simulink model "Quanser_Simulation2"  (R2019b)
settings: Solver=VariableStepAuto  StartTime=0.0  StopTime=100  RelTol=1e-3
values from neighbouring files (symbols this model uses):
  Ix = 0.0552    [ProportionalController.m]    (also in discrete1.m; discrete2.m; istr.m; proportionalTest.m = 0.0235)
  Iy = 0.0552    [ProportionalController.m]    (also in discrete1.m; discrete2.m; istr.m; proportionalTest.m = 0.0494)
  Iz = 0.11    [ProportionalController.m]    (also in discrete1.m; discrete2.m; istr.m; proportionalTest.m = 0.6121)
  K = [Ky(:,1),Kp(:,1),Kr(:,1),Ky(:,2),Kp(:,2),Kr(:,2)]    [ProportionalController.m]    (also in RLS_demo_init.m = 1; discrete1.m = 0.001; proportionalTest.m = [2.5273 0.4416 0 0 0 0)
libraries: simulink_extras x12
settings Model: Creator=YvesDaoud  LastModifiedBy=ramzih15
settings DataIOCC: ReturnWorkspaceOutputs=off
settings DebuggingCC: ArithmeticOperatorsInVariantConditions=warning
settings SFSimCC: SimUseLocalCustomCode=off  CustomCodeUndefinedFunction=UseInterfaceOnly
settings RTWCC: RTWUseLocalCustomCode=off

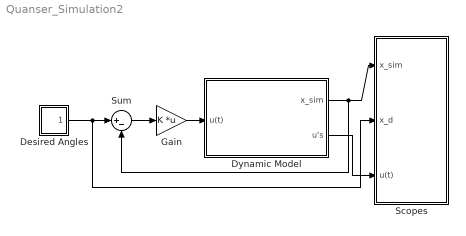
== system Quanser_Simulation2 ==
  Desired Angles : Subsystem
  Dynamic Model : Subsystem
  Gain : Gain  Gain=K  Multiplication=Matrix(K*u)
  Scopes : Subsystem
  Sum : Sum  Inputs=|+-
  wires:
  Gain/1 -> Dynamic Model/1(u(t))
  Desired Angles/1(x_d) -> Scopes/2(x_d), Sum/1
  Sum/1 -> Gain/1
  Dynamic Model/1(x_sim) -> Sum/2, Scopes/1(x_sim)
  Dynamic Model/2(u's) -> Scopes/3(u(t))

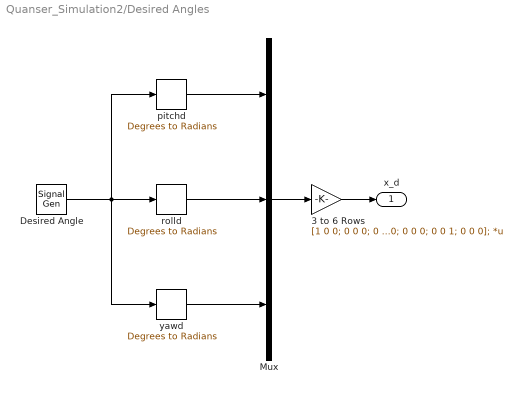
== system Quanser_Simulation2/Desired Angles ==
  3 to 6 Rows : Gain  Gain=[1 0 0; 0 0 0; 0 1 0; 0 0 0; 0 0 1; 0 0 0];  Multiplication=Matrix(K*u)
  Desired Angle : SignalGenerator  WaveForm=square  Amplitude=5  Frequency=0.05
  Mux : Mux  Inputs=3
  pitchd : simulink_extras/Transformations/Degrees to Radians
  rolld : simulink_extras/Transformations/Degrees to Radians
  yawd : simulink_extras/Transformations/Degrees to Radians
  x_d : Outport  VectorParamsAs1DForOutWhenUnconnected=off
  wires:
  3 to 6 Rows/1 -> x_d/1
  Mux/1 -> 3 to 6 Rows/1
  Desired Angle/1 -> pitchd/1, yawd/1, rolld/1
  yawd/1 -> Mux/3
  pitchd/1 -> Mux/1
  rolld/1 -> Mux/2

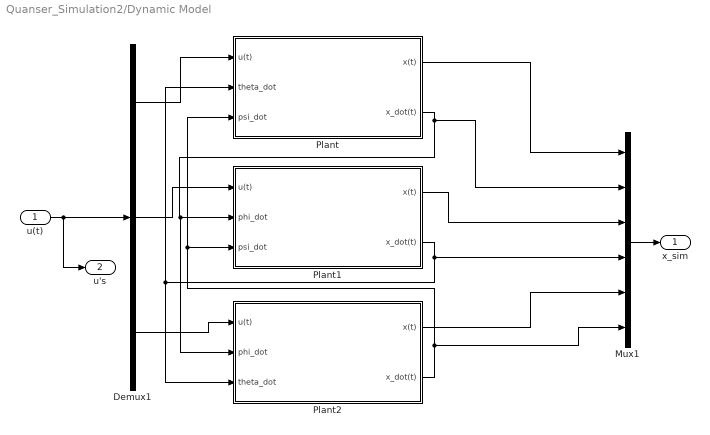
== system Quanser_Simulation2/Dynamic Model ==
  u(t) : Inport
  Demux1 : Demux  Outputs=3
  Mux1 : Mux  Inputs=6
  Plant : Subsystem
  Plant1 : Subsystem
  Plant2 : Subsystem
  x_sim : Outport  VectorParamsAs1DForOutWhenUnconnected=off
  u's : Outport  Port=2  VectorParamsAs1DForOutWhenUnconnected=off
  wires:
  Mux1/1 -> x_sim/1
  u(t)/1 -> u's/1, Demux1/1
  Demux1/1 -> Plant/1(u(t))
  Plant2/2(x_dot(t)) -> Mux1/6, Plant1/3(psi_dot), Plant/3(psi_dot)
  Plant/2(x_dot(t)) -> Mux1/2, Plant2/2(phi_dot), Plant1/2(phi_dot)
  Plant1/2(x_dot(t)) -> Mux1/4, Plant/2(theta_dot), Plant2/3(theta_dot)
  Plant/1(x(t)) -> Mux1/1
  Plant1/1(x(t)) -> Mux1/3
  Plant2/1(x(t)) -> Mux1/5
  Demux1/2 -> Plant1/1(u(t))
  Demux1/3 -> Plant2/1(u(t))

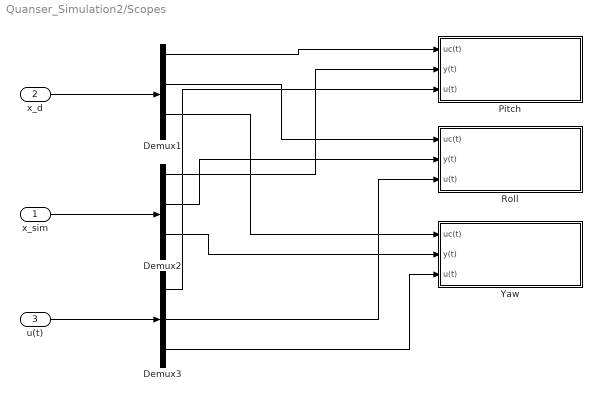
== system Quanser_Simulation2/Scopes ==
  x_sim : Inport
  x_d : Inport  Port=2
  u(t) : Inport  Port=3
  Demux1 : Demux  Outputs=6
  Demux2 : Demux  Outputs=6
  Demux3 : Demux  Outputs=3
  Pitch : Subsystem
  Roll : Subsystem
  Yaw : Subsystem
  wires:
  x_d/1 -> Demux1/1
  Demux1/1 -> Pitch/1(uc(t))
  x_sim/1 -> Demux2/1
  Demux2/1 -> Pitch/2(y(t))
  Demux1/3 -> Roll/1(uc(t))
  Demux1/5 -> Yaw/1(uc(t))
  Demux2/3 -> Roll/2(y(t))
  Demux2/5 -> Yaw/2(y(t))
  u(t)/1 -> Demux3/1
  Demux3/1 -> Pitch/3(u(t))
  Demux3/2 -> Roll/3(u(t))
  Demux3/3 -> Yaw/3(u(t))

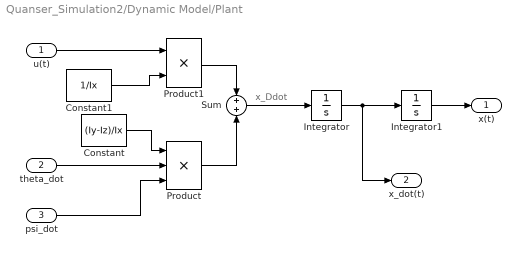
== system Quanser_Simulation2/Dynamic Model/Plant ==
  note: x_Ddot
  u(t) : Inport
  theta_dot : Inport  Port=2
  psi_dot : Inport  Port=3
  Constant : Constant  Value=(Iy-Iz)/Ix
  Constant1 : Constant  Value=1/Ix
  Integrator : Integrator
  Integrator1 : Integrator
  Product : Product  Inputs=3
  Product1 : Product
  Sum : Sum  Inputs=+|+
  x(t) : Outport  VectorParamsAs1DForOutWhenUnconnected=off
  x_dot(t) : Outport  Port=2  VectorParamsAs1DForOutWhenUnconnected=off
  wires:
  Constant/1 -> Product/1
  theta_dot/1 -> Product/2
  psi_dot/1 -> Product/3
  u(t)/1 -> Product1/1
  Constant1/1 -> Product1/2
  Product/1 -> Sum/2
  Product1/1 -> Sum/1
  Sum/1 -> Integrator/1
  Integrator/1 -> x_dot(t)/1, Integrator1/1
  Integrator1/1 -> x(t)/1

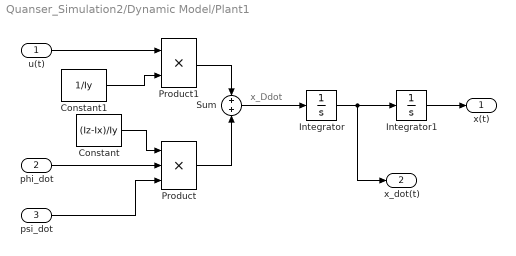
== system Quanser_Simulation2/Dynamic Model/Plant1 ==
  note: x_Ddot
  u(t) : Inport
  phi_dot : Inport  Port=2
  psi_dot : Inport  Port=3
  Constant : Constant  Value=(Iz-Ix)/Iy
  Constant1 : Constant  Value=1/Iy
  Integrator : Integrator
  Integrator1 : Integrator
  Product : Product  Inputs=3
  Product1 : Product
  Sum : Sum  Inputs=+|+
  x(t) : Outport  VectorParamsAs1DForOutWhenUnconnected=off
  x_dot(t) : Outport  Port=2  VectorParamsAs1DForOutWhenUnconnected=off
  wires:
  Integrator1/1 -> x(t)/1
  Integrator/1 -> Integrator1/1, x_dot(t)/1
  Sum/1 -> Integrator/1
  Product1/1 -> Sum/1
  Product/1 -> Sum/2
  Constant1/1 -> Product1/2
  u(t)/1 -> Product1/1
  psi_dot/1 -> Product/3
  phi_dot/1 -> Product/2
  Constant/1 -> Product/1

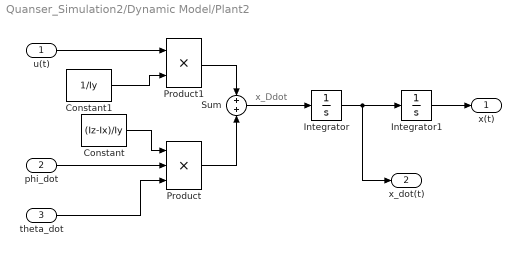
== system Quanser_Simulation2/Dynamic Model/Plant2 ==
  note: x_Ddot
  u(t) : Inport
  phi_dot : Inport  Port=2
  theta_dot : Inport  Port=3
  Constant : Constant  Value=(Iz-Ix)/Iy
  Constant1 : Constant  Value=1/Iy
  Integrator : Integrator
  Integrator1 : Integrator
  Product : Product  Inputs=3
  Product1 : Product
  Sum : Sum  Inputs=+|+
  x(t) : Outport  VectorParamsAs1DForOutWhenUnconnected=off
  x_dot(t) : Outport  Port=2  VectorParamsAs1DForOutWhenUnconnected=off
  wires:
  Constant/1 -> Product/1
  phi_dot/1 -> Product/2
  theta_dot/1 -> Product/3
  u(t)/1 -> Product1/1
  Constant1/1 -> Product1/2
  Product/1 -> Sum/2
  Product1/1 -> Sum/1
  Sum/1 -> Integrator/1
  Integrator/1 -> x_dot(t)/1, Integrator1/1
  Integrator1/1 -> x(t)/1

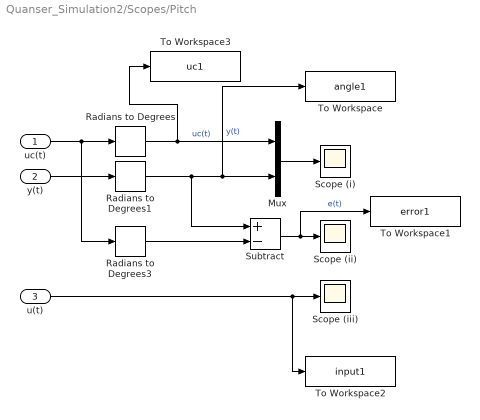
== system Quanser_Simulation2/Scopes/Pitch ==
  uc(t) : Inport
  y(t) : Inport  Port=2
  u(t) : Inport  Port=3
  Mux : Mux  Inputs=2
  Radians to Degrees : simulink_extras/Transformations/Radians to Degrees
  Radians to Degrees1 : simulink_extras/Transformations/Radians to Degrees
  Radians to Degrees3 : simulink_extras/Transformations/Radians to Degrees
  Scope (i) : Scope
  Scope (ii) : Scope
  Scope (iii) : Scope
  Subtract : Sum  Inputs=+-
  To Workspace : ToWorkspace  VariableName=angle1  SampleTime=-1
  To Workspace1 : ToWorkspace  VariableName=error1  SampleTime=-1
  To Workspace2 : ToWorkspace  VariableName=input1  SampleTime=-1
  To Workspace3 : ToWorkspace  VariableName=uc1  SampleTime=-1
  wires:
  Mux/1 -> Scope (i)/1
  Subtract/1 -> To Workspace1/1, Scope (ii)/1  "e(t)"
  y(t)/1 -> Radians to Degrees1/1
  uc(t)/1 -> Radians to Degrees3/1, Radians to Degrees/1
  u(t)/1 -> To Workspace2/1, Scope (iii)/1
  Radians to Degrees/1 -> To Workspace3/1, Mux/1  "uc(t)"
  Radians to Degrees1/1 -> Subtract/1, To Workspace/1, Mux/2  "y(t)"
  Radians to Degrees3/1 -> Subtract/2

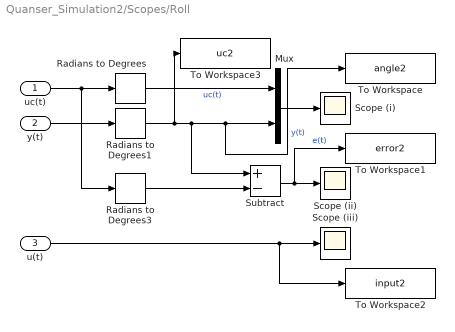
== system Quanser_Simulation2/Scopes/Roll ==
  uc(t) : Inport
  y(t) : Inport  Port=2
  u(t) : Inport  Port=3
  Mux : Mux  Inputs=2
  Radians to Degrees : simulink_extras/Transformations/Radians to Degrees
  Radians to Degrees1 : simulink_extras/Transformations/Radians to Degrees
  Radians to Degrees3 : simulink_extras/Transformations/Radians to Degrees
  Scope (i) : Scope
  Scope (ii) : Scope
  Scope (iii) : Scope
  Subtract : Sum  Inputs=+-
  To Workspace : ToWorkspace  VariableName=angle2  SampleTime=-1
  To Workspace1 : ToWorkspace  VariableName=error2  SampleTime=-1
  To Workspace2 : ToWorkspace  VariableName=input2  SampleTime=-1
  To Workspace3 : ToWorkspace  VariableName=uc2  SampleTime=-1
  wires:
  Radians to Degrees3/1 -> Subtract/2
  Radians to Degrees1/1 -> To Workspace3/1, To Workspace/1, Mux/2, Subtract/1  "y(t)"
  Radians to Degrees/1 -> Mux/1  "uc(t)"
  uc(t)/1 -> Radians to Degrees/1, Radians to Degrees3/1
  y(t)/1 -> Radians to Degrees1/1
  Subtract/1 -> To Workspace1/1, Scope (ii)/1  "e(t)"
  Mux/1 -> Scope (i)/1
  u(t)/1 -> To Workspace2/1, Scope (iii)/1

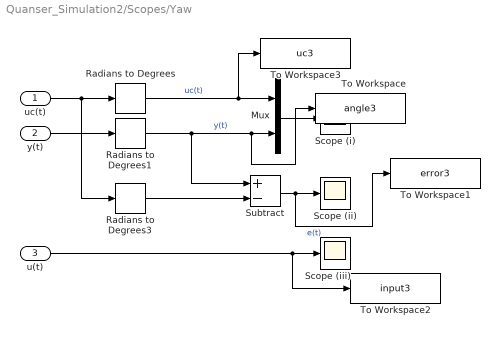
== system Quanser_Simulation2/Scopes/Yaw ==
  uc(t) : Inport
  y(t) : Inport  Port=2
  u(t) : Inport  Port=3
  Mux : Mux  Inputs=2
  Radians to Degrees : simulink_extras/Transformations/Radians to Degrees
  Radians to Degrees1 : simulink_extras/Transformations/Radians to Degrees
  Radians to Degrees3 : simulink_extras/Transformations/Radians to Degrees
  Scope (i) : Scope
  Scope (ii) : Scope
  Scope (iii) : Scope
  Subtract : Sum  Inputs=+-
  To Workspace : ToWorkspace  VariableName=angle3  SampleTime=-1
  To Workspace1 : ToWorkspace  VariableName=error3  SampleTime=-1
  To Workspace2 : ToWorkspace  VariableName=input3  SampleTime=-1
  To Workspace3 : ToWorkspace  VariableName=uc3  SampleTime=-1
  wires:
  Mux/1 -> Scope (i)/1
  Subtract/1 -> To Workspace1/1, Scope (ii)/1  "e(t)"
  y(t)/1 -> Radians to Degrees1/1
  uc(t)/1 -> Radians to Degrees3/1, Radians to Degrees/1
  u(t)/1 -> To Workspace2/1, Scope (iii)/1
  Radians to Degrees/1 -> To Workspace3/1, Mux/1  "uc(t)"
  Radians to Degrees1/1 -> Subtract/1, To Workspace/1, Mux/2  "y(t)"
  Radians to Degrees3/1 -> Subtract/2
